simulink model "neuronchainv5"  (Simulink 7.6)
settings: Solver=ode45  StartTime=0.0  StopTime=200  RelTol=1e-3
values from neighbouring files (symbols this model uses):
  alpha = 0.8    [excneuroninit.m]
  beta = 0.05    [excneuroninit.m]
  inittime = 0.1    [excneuroninit.m]
  sensoryamp = 0.5    [excneuroninit.m]
  sigslopef = 1    [excneuroninit.m]
  sigslopei = 3    [excneuroninit.m]
  tau_s = 5    [excneuroninit.m]
libraries: simulink x500, neuronpoolibv3 x3
(part 7 of 18)

== system neuronchainv5/Hebbconp5/44 ==
  ui : Inport
  uj : Inport  Port=2
  Sij : Inport  Port=3
  1_over_taus : Gain  Gain=1/tau_s
  Clock : Clock
      settings: Decimation=10
  Constant : Constant  Value=alpha
  Constant3 : Constant  Value=inittime
  Integrator : Integrator
  Product : Product  Inputs=3  RndMeth=Zero
  Product1 : Product  RndMeth=Zero
  Sum : Sum  Inputs=|+-
  Sum1 : Sum  Inputs=|+-
  Sum2 : Sum  Inputs=+-|
  Switch1 : Switch  Criteria=u2 > Threshold
  beta : Gain  Gain=beta
  f(ui) : Subsystem  TreatAsAtomicUnit=on  mask{slope=sigslopef, offset=0.5}
      mask help: Created by Han, Cheol
      mask Display: plot([10 15 20 25 30 35 40 45 50], [0 0.01 0.1 0.2 0.5 0.8 0.9 0.99 1])
  f(uj) : Subsystem  TreatAsAtomicUnit=on  mask{slope=sigslopef, offset=0.5}
      mask help: Created by Han, Cheol
      mask Display: plot([10 15 20 25 30 35 40 45 50], [0 0.01 0.1 0.2 0.5 0.8 0.9 0.99 1])
  h(ui) : Subsystem  TreatAsAtomicUnit=on  mask{slope=sigslopei, offset=0.5}
      mask help: Created by Han, Cheol
      mask Display: plot([10 15 20 25 30 35 40 45 50], [0 0.01 0.1 0.2 0.5 0.8 0.9 0.99 1])
  Out1 : Outport
  wires:
  ui/1 -> h(ui)/1(x), f(ui)/1(x)
  uj/1 -> f(uj)/1(x)
  f(ui)/1(y) -> Product/1
  f(uj)/1(y) -> Product/2
  Constant/1 -> Product/3
  Product/1 -> Sum/1
  Sum/1 -> Product1/2
  h(ui)/1(y) -> Product1/1
  Product1/1 -> Sum1/1
  beta/1 -> Sum1/2
  Sum1/1 -> 1_over_taus/1
  1_over_taus/1 -> Integrator/1
  Integrator/1 -> Switch1/1, Sum/2
  Sum2/1 -> Switch1/2
  Clock/1 -> Sum2/1
  Constant3/1 -> Sum2/2
  Switch1/1 -> beta/1, Out1/1
  Sij/1 -> Switch1/3

== system neuronchainv5/Hebbconp5/45 ==
  ui : Inport
  uj : Inport  Port=2
  Sij : Inport  Port=3
  1_over_taus : Gain  Gain=1/tau_s
  Clock : Clock
      settings: Decimation=10
  Constant : Constant  Value=alpha
  Constant3 : Constant  Value=inittime
  Integrator : Integrator
  Product : Product  Inputs=3  RndMeth=Zero
  Product1 : Product  RndMeth=Zero
  Sum : Sum  Inputs=|+-
  Sum1 : Sum  Inputs=|+-
  Sum2 : Sum  Inputs=+-|
  Switch1 : Switch  Criteria=u2 > Threshold
  beta : Gain  Gain=beta
  f(ui) : Subsystem  TreatAsAtomicUnit=on  mask{slope=sigslopef, offset=0.5}
      mask help: Created by Han, Cheol
      mask Display: plot([10 15 20 25 30 35 40 45 50], [0 0.01 0.1 0.2 0.5 0.8 0.9 0.99 1])
  f(uj) : Subsystem  TreatAsAtomicUnit=on  mask{slope=sigslopef, offset=0.5}
      mask help: Created by Han, Cheol
      mask Display: plot([10 15 20 25 30 35 40 45 50], [0 0.01 0.1 0.2 0.5 0.8 0.9 0.99 1])
  h(ui) : Subsystem  TreatAsAtomicUnit=on  mask{slope=sigslopei, offset=0.5}
      mask help: Created by Han, Cheol
      mask Display: plot([10 15 20 25 30 35 40 45 50], [0 0.01 0.1 0.2 0.5 0.8 0.9 0.99 1])
  Out1 : Outport
  wires:
  ui/1 -> h(ui)/1(x), f(ui)/1(x)
  uj/1 -> f(uj)/1(x)
  f(ui)/1(y) -> Product/1
  f(uj)/1(y) -> Product/2
  Constant/1 -> Product/3
  Product/1 -> Sum/1
  Sum/1 -> Product1/2
  h(ui)/1(y) -> Product1/1
  Product1/1 -> Sum1/1
  beta/1 -> Sum1/2
  Sum1/1 -> 1_over_taus/1
  1_over_taus/1 -> Integrator/1
  Integrator/1 -> Switch1/1, Sum/2
  Sum2/1 -> Switch1/2
  Clock/1 -> Sum2/1
  Constant3/1 -> Sum2/2
  Switch1/1 -> beta/1, Out1/1
  Sij/1 -> Switch1/3

== system neuronchainv5/Hebbconp5/5 ==
  ui : Inport
  uj : Inport  Port=2
  Sij : Inport  Port=3
  1_over_taus : Gain  Gain=1/tau_s
  Clock : Clock
      settings: Decimation=10
  Constant : Constant  Value=alpha
  Constant3 : Constant  Value=inittime
  Integrator : Integrator
  Product : Product  Inputs=3  RndMeth=Zero
  Product1 : Product  RndMeth=Zero
  Sum : Sum  Inputs=|+-
  Sum1 : Sum  Inputs=|+-
  Sum2 : Sum  Inputs=+-|
  Switch1 : Switch  Criteria=u2 > Threshold
  beta : Gain  Gain=beta
  f(ui) : Subsystem  TreatAsAtomicUnit=on  mask{slope=sigslopef, offset=0.5}
      mask help: Created by Han, Cheol
      mask Display: plot([10 15 20 25 30 35 40 45 50], [0 0.01 0.1 0.2 0.5 0.8 0.9 0.99 1])
  f(uj) : Subsystem  TreatAsAtomicUnit=on  mask{slope=sigslopef, offset=0.5}
      mask help: Created by Han, Cheol
      mask Display: plot([10 15 20 25 30 35 40 45 50], [0 0.01 0.1 0.2 0.5 0.8 0.9 0.99 1])
  h(ui) : Subsystem  TreatAsAtomicUnit=on  mask{slope=sigslopei, offset=0.5}
      mask help: Created by Han, Cheol
      mask Display: plot([10 15 20 25 30 35 40 45 50], [0 0.01 0.1 0.2 0.5 0.8 0.9 0.99 1])
  Out1 : Outport
  wires:
  ui/1 -> h(ui)/1(x), f(ui)/1(x)
  uj/1 -> f(uj)/1(x)
  f(ui)/1(y) -> Product/1
  f(uj)/1(y) -> Product/2
  Constant/1 -> Product/3
  Product/1 -> Sum/1
  Sum/1 -> Product1/2
  h(ui)/1(y) -> Product1/1
  Product1/1 -> Sum1/1
  beta/1 -> Sum1/2
  Sum1/1 -> 1_over_taus/1
  1_over_taus/1 -> Integrator/1
  Integrator/1 -> Switch1/1, Sum/2
  Sum2/1 -> Switch1/2
  Clock/1 -> Sum2/1
  Constant3/1 -> Sum2/2
  Switch1/1 -> beta/1, Out1/1
  Sij/1 -> Switch1/3

== system neuronchainv5/Hebbconp5/f(uj)1 ==
  x : Inport
  Constant : Constant  Value=offset
  Constant1 : Constant  Value=slope
  Constant2 : Constant
  Gain : Gain  Gain=-1  SaturateOnIntegerOverflow=on  OutDataTypeStr=Inherit: Same as input  ParamDataTypeStr=Inherit: Same as input
  Math Function : Math  SaturateOnIntegerOverflow=on
  Math Function1 : Math  Operator=reciprocal  SaturateOnIntegerOverflow=on
  Model Info : simulink/Model-Wide Utilities/Model Info  SystemSampleTime=-1  InitialBlockCM=None  BlockCM=None  Frame=on  DisplayStringWithTags=|  HorizontalTextAlignment=Center  LeftAlignmentValue=0.5  SourceBlockDiagram=neuronchainv5  TagMaxNumber=20
      | Model Info
      | %<Creator> Han, Cheol
  Product : Product  SaturateOnIntegerOverflow=on  OutDataTypeStr=Inherit: Same as first input
  Sum : Sum  Inputs=+-  SaturateOnIntegerOverflow=on
  Sum1 : Sum  SaturateOnIntegerOverflow=on
  y : Outport  InitialOutput=0
  wires:
  x/1 -> Sum/1
  Constant/1 -> Sum/2
  Sum/1 -> Product/1
  Constant1/1 -> Product/2
  Product/1 -> Gain/1
  Gain/1 -> Math Function/1
  Math Function/1 -> Sum1/1
  Constant2/1 -> Sum1/2
  Sum1/1 -> Math Function1/1
  Math Function1/1 -> y/1

== system neuronchainv5/Hebbconp5/f(uj)2 ==
  x : Inport
  Constant : Constant  Value=offset
  Constant1 : Constant  Value=slope
  Constant2 : Constant
  Gain : Gain  Gain=-1  SaturateOnIntegerOverflow=on  OutDataTypeStr=Inherit: Same as input  ParamDataTypeStr=Inherit: Same as input
  Math Function : Math  SaturateOnIntegerOverflow=on
  Math Function1 : Math  Operator=reciprocal  SaturateOnIntegerOverflow=on
  Model Info : simulink/Model-Wide Utilities/Model Info  SystemSampleTime=-1  InitialBlockCM=None  BlockCM=None  Frame=on  DisplayStringWithTags=|  HorizontalTextAlignment=Center  LeftAlignmentValue=0.5  SourceBlockDiagram=neuronchainv5  TagMaxNumber=20
      | Model Info
      | %<Creator> Han, Cheol
  Product : Product  SaturateOnIntegerOverflow=on  OutDataTypeStr=Inherit: Same as first input
  Sum : Sum  Inputs=+-  SaturateOnIntegerOverflow=on
  Sum1 : Sum  SaturateOnIntegerOverflow=on
  y : Outport  InitialOutput=0
  wires:
  x/1 -> Sum/1
  Constant/1 -> Sum/2
  Sum/1 -> Product/1
  Constant1/1 -> Product/2
  Product/1 -> Gain/1
  Gain/1 -> Math Function/1
  Math Function/1 -> Sum1/1
  Constant2/1 -> Sum1/2
  Sum1/1 -> Math Function1/1
  Math Function1/1 -> y/1

== system neuronchainv5/Hebbconp5/f(uj)3 ==
  x : Inport
  Constant : Constant  Value=offset
  Constant1 : Constant  Value=slope
  Constant2 : Constant
  Gain : Gain  Gain=-1  SaturateOnIntegerOverflow=on  OutDataTypeStr=Inherit: Same as input  ParamDataTypeStr=Inherit: Same as input
  Math Function : Math  SaturateOnIntegerOverflow=on
  Math Function1 : Math  Operator=reciprocal  SaturateOnIntegerOverflow=on
  Model Info : simulink/Model-Wide Utilities/Model Info  SystemSampleTime=-1  InitialBlockCM=None  BlockCM=None  Frame=on  DisplayStringWithTags=|  HorizontalTextAlignment=Center  LeftAlignmentValue=0.5  SourceBlockDiagram=neuronchainv5  TagMaxNumber=20
      | Model Info
      | %<Creator> Han, Cheol
  Product : Product  SaturateOnIntegerOverflow=on  OutDataTypeStr=Inherit: Same as first input
  Sum : Sum  Inputs=+-  SaturateOnIntegerOverflow=on
  Sum1 : Sum  SaturateOnIntegerOverflow=on
  y : Outport  InitialOutput=0
  wires:
  x/1 -> Sum/1
  Constant/1 -> Sum/2
  Sum/1 -> Product/1
  Constant1/1 -> Product/2
  Product/1 -> Gain/1
  Gain/1 -> Math Function/1
  Math Function/1 -> Sum1/1
  Constant2/1 -> Sum1/2
  Sum1/1 -> Math Function1/1
  Math Function1/1 -> y/1

== system neuronchainv5/Hebbconp5/f(uj)4 ==
  x : Inport
  Constant : Constant  Value=offset
  Constant1 : Constant  Value=slope
  Constant2 : Constant
  Gain : Gain  Gain=-1  SaturateOnIntegerOverflow=on  OutDataTypeStr=Inherit: Same as input  ParamDataTypeStr=Inherit: Same as input
  Math Function : Math  SaturateOnIntegerOverflow=on
  Math Function1 : Math  Operator=reciprocal  SaturateOnIntegerOverflow=on
  Model Info : simulink/Model-Wide Utilities/Model Info  SystemSampleTime=-1  InitialBlockCM=None  BlockCM=None  Frame=on  DisplayStringWithTags=|  HorizontalTextAlignment=Center  LeftAlignmentValue=0.5  SourceBlockDiagram=neuronchainv5  TagMaxNumber=20
      | Model Info
      | %<Creator> Han, Cheol
  Product : Product  SaturateOnIntegerOverflow=on  OutDataTypeStr=Inherit: Same as first input
  Sum : Sum  Inputs=+-  SaturateOnIntegerOverflow=on
  Sum1 : Sum  SaturateOnIntegerOverflow=on
  y : Outport  InitialOutput=0
  wires:
  x/1 -> Sum/1
  Constant/1 -> Sum/2
  Sum/1 -> Product/1
  Constant1/1 -> Product/2
  Product/1 -> Gain/1
  Gain/1 -> Math Function/1
  Math Function/1 -> Sum1/1
  Constant2/1 -> Sum1/2
  Sum1/1 -> Math Function1/1
  Math Function1/1 -> y/1

== system neuronchainv5/Hebbconp5/f(uj)5 ==
  x : Inport
  Constant : Constant  Value=offset
  Constant1 : Constant  Value=slope
  Constant2 : Constant
  Gain : Gain  Gain=-1  SaturateOnIntegerOverflow=on  OutDataTypeStr=Inherit: Same as input  ParamDataTypeStr=Inherit: Same as input
  Math Function : Math  SaturateOnIntegerOverflow=on
  Math Function1 : Math  Operator=reciprocal  SaturateOnIntegerOverflow=on
  Model Info : simulink/Model-Wide Utilities/Model Info  SystemSampleTime=-1  InitialBlockCM=None  BlockCM=None  Frame=on  DisplayStringWithTags=|  HorizontalTextAlignment=Center  LeftAlignmentValue=0.5  SourceBlockDiagram=neuronchainv5  TagMaxNumber=20
      | Model Info
      | %<Creator> Han, Cheol
  Product : Product  SaturateOnIntegerOverflow=on  OutDataTypeStr=Inherit: Same as first input
  Sum : Sum  Inputs=+-  SaturateOnIntegerOverflow=on
  Sum1 : Sum  SaturateOnIntegerOverflow=on
  y : Outport  InitialOutput=0
  wires:
  x/1 -> Sum/1
  Constant/1 -> Sum/2
  Sum/1 -> Product/1
  Constant1/1 -> Product/2
  Product/1 -> Gain/1
  Gain/1 -> Math Function/1
  Math Function/1 -> Sum1/1
  Constant2/1 -> Sum1/2
  Sum1/1 -> Math Function1/1
  Math Function1/1 -> y/1

== system neuronchainv5/Subsystem/motoract vis inputs ==
  Mux : Mux  Inputs=5
  Mux1 : Mux  Inputs=5
  Subsystem : Subsystem
  Subsystem1 : Subsystem
  Subsystem2 : Subsystem
  Subsystem3 : Subsystem
  Subsystem4 : Subsystem
  Out1 : Outport
  Out2 : Outport  Port=2
  wires:
  Subsystem/1(Out1) -> Mux/1
  Subsystem3/1(Out1) -> Mux/4
  Subsystem/2(Out2) -> Mux1/1
  Subsystem2/2(Out2) -> Mux1/3
  Subsystem3/2(Out2) -> Mux1/4
  Mux/1 -> Out1/1
  Mux1/1 -> Out2/1
  Subsystem1/2(Out2) -> Mux1/2
  Subsystem1/1(Out1) -> Mux/2
  Subsystem2/1(Out1) -> Mux/3
  Subsystem4/2(Out2) -> Mux1/5
  Subsystem4/1(Out1) -> Mux/5

== system neuronchainv5/Hebbconp/ /f(ui) ==
  x : Inport
  Constant : Constant  Value=offset
  Constant1 : Constant  Value=slope
  Constant2 : Constant
  Gain : Gain  Gain=-1  SaturateOnIntegerOverflow=on  OutDataTypeStr=Inherit: Same as input  ParamDataTypeStr=Inherit: Same as input
  Math Function : Math  SaturateOnIntegerOverflow=on
  Math Function1 : Math  Operator=reciprocal  SaturateOnIntegerOverflow=on
  Model Info : simulink/Model-Wide Utilities/Model Info  SystemSampleTime=-1  InitialBlockCM=None  BlockCM=None  Frame=on  DisplayStringWithTags=|  HorizontalTextAlignment=Center  LeftAlignmentValue=0.5  SourceBlockDiagram=neuronchainv5  TagMaxNumber=20
      | Model Info
      | %<Creator> Han, Cheol
  Product : Product  SaturateOnIntegerOverflow=on  OutDataTypeStr=Inherit: Same as first input
  Sum : Sum  Inputs=+-  SaturateOnIntegerOverflow=on
  Sum1 : Sum  SaturateOnIntegerOverflow=on
  y : Outport  InitialOutput=0
  wires:
  x/1 -> Sum/1
  Constant/1 -> Sum/2
  Sum/1 -> Product/1
  Constant1/1 -> Product/2
  Product/1 -> Gain/1
  Gain/1 -> Math Function/1
  Math Function/1 -> Sum1/1
  Constant2/1 -> Sum1/2
  Sum1/1 -> Math Function1/1
  Math Function1/1 -> y/1

== system neuronchainv5/Hebbconp/ /f(uj) ==
  x : Inport
  Constant : Constant  Value=offset
  Constant1 : Constant  Value=slope
  Constant2 : Constant
  Gain : Gain  Gain=-1  SaturateOnIntegerOverflow=on  OutDataTypeStr=Inherit: Same as input  ParamDataTypeStr=Inherit: Same as input
  Math Function : Math  SaturateOnIntegerOverflow=on
  Math Function1 : Math  Operator=reciprocal  SaturateOnIntegerOverflow=on
  Model Info : simulink/Model-Wide Utilities/Model Info  SystemSampleTime=-1  InitialBlockCM=None  BlockCM=None  Frame=on  DisplayStringWithTags=|  HorizontalTextAlignment=Center  LeftAlignmentValue=0.5  SourceBlockDiagram=neuronchainv5  TagMaxNumber=20
      | Model Info
      | %<Creator> Han, Cheol
  Product : Product  SaturateOnIntegerOverflow=on  OutDataTypeStr=Inherit: Same as first input
  Sum : Sum  Inputs=+-  SaturateOnIntegerOverflow=on
  Sum1 : Sum  SaturateOnIntegerOverflow=on
  y : Outport  InitialOutput=0
  wires:
  x/1 -> Sum/1
  Constant/1 -> Sum/2
  Sum/1 -> Product/1
  Constant1/1 -> Product/2
  Product/1 -> Gain/1
  Gain/1 -> Math Function/1
  Math Function/1 -> Sum1/1
  Constant2/1 -> Sum1/2
  Sum1/1 -> Math Function1/1
  Math Function1/1 -> y/1

== system neuronchainv5/Hebbconp/ /h(ui) ==
  x : Inport
  Constant : Constant  Value=offset
  Constant1 : Constant  Value=slope
  Constant2 : Constant
  Gain : Gain  Gain=-1  SaturateOnIntegerOverflow=on  OutDataTypeStr=Inherit: Same as input  ParamDataTypeStr=Inherit: Same as input
  Math Function : Math  SaturateOnIntegerOverflow=on
  Math Function1 : Math  Operator=reciprocal  SaturateOnIntegerOverflow=on
  Model Info : simulink/Model-Wide Utilities/Model Info  SystemSampleTime=-1  InitialBlockCM=None  BlockCM=None  Frame=on  DisplayStringWithTags=|  HorizontalTextAlignment=Center  LeftAlignmentValue=0.5  SourceBlockDiagram=neuronchainv5  TagMaxNumber=20
      | Model Info
      | %<Creator> Han, Cheol
  Product : Product  SaturateOnIntegerOverflow=on  OutDataTypeStr=Inherit: Same as first input
  Sum : Sum  Inputs=+-  SaturateOnIntegerOverflow=on
  Sum1 : Sum  SaturateOnIntegerOverflow=on
  y : Outport  InitialOutput=0
  wires:
  x/1 -> Sum/1
  Constant/1 -> Sum/2
  Sum/1 -> Product/1
  Constant1/1 -> Product/2
  Product/1 -> Gain/1
  Gain/1 -> Math Function/1
  Math Function/1 -> Sum1/1
  Constant2/1 -> Sum1/2
  Sum1/1 -> Math Function1/1
  Math Function1/1 -> y/1

== system neuronchainv5/Hebbconp/ 2/f(ui) ==
  x : Inport
  Constant : Constant  Value=offset
  Constant1 : Constant  Value=slope
  Constant2 : Constant
  Gain : Gain  Gain=-1  SaturateOnIntegerOverflow=on  OutDataTypeStr=Inherit: Same as input  ParamDataTypeStr=Inherit: Same as input
  Math Function : Math  SaturateOnIntegerOverflow=on
  Math Function1 : Math  Operator=reciprocal  SaturateOnIntegerOverflow=on
  Model Info : simulink/Model-Wide Utilities/Model Info  SystemSampleTime=-1  InitialBlockCM=None  BlockCM=None  Frame=on  DisplayStringWithTags=|  HorizontalTextAlignment=Center  LeftAlignmentValue=0.5  SourceBlockDiagram=neuronchainv5  TagMaxNumber=20
      | Model Info
      | %<Creator> Han, Cheol
  Product : Product  SaturateOnIntegerOverflow=on  OutDataTypeStr=Inherit: Same as first input
  Sum : Sum  Inputs=+-  SaturateOnIntegerOverflow=on
  Sum1 : Sum  SaturateOnIntegerOverflow=on
  y : Outport  InitialOutput=0
  wires:
  x/1 -> Sum/1
  Constant/1 -> Sum/2
  Sum/1 -> Product/1
  Constant1/1 -> Product/2
  Product/1 -> Gain/1
  Gain/1 -> Math Function/1
  Math Function/1 -> Sum1/1
  Constant2/1 -> Sum1/2
  Sum1/1 -> Math Function1/1
  Math Function1/1 -> y/1

== system neuronchainv5/Hebbconp/ 2/f(uj) ==
  x : Inport
  Constant : Constant  Value=offset
  Constant1 : Constant  Value=slope
  Constant2 : Constant
  Gain : Gain  Gain=-1  SaturateOnIntegerOverflow=on  OutDataTypeStr=Inherit: Same as input  ParamDataTypeStr=Inherit: Same as input
  Math Function : Math  SaturateOnIntegerOverflow=on
  Math Function1 : Math  Operator=reciprocal  SaturateOnIntegerOverflow=on
  Model Info : simulink/Model-Wide Utilities/Model Info  SystemSampleTime=-1  InitialBlockCM=None  BlockCM=None  Frame=on  DisplayStringWithTags=|  HorizontalTextAlignment=Center  LeftAlignmentValue=0.5  SourceBlockDiagram=neuronchainv5  TagMaxNumber=20
      | Model Info
      | %<Creator> Han, Cheol
  Product : Product  SaturateOnIntegerOverflow=on  OutDataTypeStr=Inherit: Same as first input
  Sum : Sum  Inputs=+-  SaturateOnIntegerOverflow=on
  Sum1 : Sum  SaturateOnIntegerOverflow=on
  y : Outport  InitialOutput=0
  wires:
  x/1 -> Sum/1
  Constant/1 -> Sum/2
  Sum/1 -> Product/1
  Constant1/1 -> Product/2
  Product/1 -> Gain/1
  Gain/1 -> Math Function/1
  Math Function/1 -> Sum1/1
  Constant2/1 -> Sum1/2
  Sum1/1 -> Math Function1/1
  Math Function1/1 -> y/1

== system neuronchainv5/Hebbconp/ 2/h(ui) ==
  x : Inport
  Constant : Constant  Value=offset
  Constant1 : Constant  Value=slope
  Constant2 : Constant
  Gain : Gain  Gain=-1  SaturateOnIntegerOverflow=on  OutDataTypeStr=Inherit: Same as input  ParamDataTypeStr=Inherit: Same as input
  Math Function : Math  SaturateOnIntegerOverflow=on
  Math Function1 : Math  Operator=reciprocal  SaturateOnIntegerOverflow=on
  Model Info : simulink/Model-Wide Utilities/Model Info  SystemSampleTime=-1  InitialBlockCM=None  BlockCM=None  Frame=on  DisplayStringWithTags=|  HorizontalTextAlignment=Center  LeftAlignmentValue=0.5  SourceBlockDiagram=neuronchainv5  TagMaxNumber=20
      | Model Info
      | %<Creator> Han, Cheol
  Product : Product  SaturateOnIntegerOverflow=on  OutDataTypeStr=Inherit: Same as first input
  Sum : Sum  Inputs=+-  SaturateOnIntegerOverflow=on
  Sum1 : Sum  SaturateOnIntegerOverflow=on
  y : Outport  InitialOutput=0
  wires:
  x/1 -> Sum/1
  Constant/1 -> Sum/2
  Sum/1 -> Product/1
  Constant1/1 -> Product/2
  Product/1 -> Gain/1
  Gain/1 -> Math Function/1
  Math Function/1 -> Sum1/1
  Constant2/1 -> Sum1/2
  Sum1/1 -> Math Function1/1
  Math Function1/1 -> y/1

== system neuronchainv5/Hebbconp/11/f(ui) ==
  x : Inport
  Constant : Constant  Value=offset
  Constant1 : Constant  Value=slope
  Constant2 : Constant
  Gain : Gain  Gain=-1  SaturateOnIntegerOverflow=on  OutDataTypeStr=Inherit: Same as input  ParamDataTypeStr=Inherit: Same as input
  Math Function : Math  SaturateOnIntegerOverflow=on
  Math Function1 : Math  Operator=reciprocal  SaturateOnIntegerOverflow=on
  Model Info : simulink/Model-Wide Utilities/Model Info  SystemSampleTime=-1  InitialBlockCM=None  BlockCM=None  Frame=on  DisplayStringWithTags=|  HorizontalTextAlignment=Center  LeftAlignmentValue=0.5  SourceBlockDiagram=neuronchainv5  TagMaxNumber=20
      | Model Info
      | %<Creator> Han, Cheol
  Product : Product  SaturateOnIntegerOverflow=on  OutDataTypeStr=Inherit: Same as first input
  Sum : Sum  Inputs=+-  SaturateOnIntegerOverflow=on
  Sum1 : Sum  SaturateOnIntegerOverflow=on
  y : Outport  InitialOutput=0
  wires:
  x/1 -> Sum/1
  Constant/1 -> Sum/2
  Sum/1 -> Product/1
  Constant1/1 -> Product/2
  Product/1 -> Gain/1
  Gain/1 -> Math Function/1
  Math Function/1 -> Sum1/1
  Constant2/1 -> Sum1/2
  Sum1/1 -> Math Function1/1
  Math Function1/1 -> y/1

== system neuronchainv5/Hebbconp/11/f(uj) ==
  x : Inport
  Constant : Constant  Value=offset
  Constant1 : Constant  Value=slope
  Constant2 : Constant
  Gain : Gain  Gain=-1  SaturateOnIntegerOverflow=on  OutDataTypeStr=Inherit: Same as input  ParamDataTypeStr=Inherit: Same as input
  Math Function : Math  SaturateOnIntegerOverflow=on
  Math Function1 : Math  Operator=reciprocal  SaturateOnIntegerOverflow=on
  Model Info : simulink/Model-Wide Utilities/Model Info  SystemSampleTime=-1  InitialBlockCM=None  BlockCM=None  Frame=on  DisplayStringWithTags=|  HorizontalTextAlignment=Center  LeftAlignmentValue=0.5  SourceBlockDiagram=neuronchainv5  TagMaxNumber=20
      | Model Info
      | %<Creator> Han, Cheol
  Product : Product  SaturateOnIntegerOverflow=on  OutDataTypeStr=Inherit: Same as first input
  Sum : Sum  Inputs=+-  SaturateOnIntegerOverflow=on
  Sum1 : Sum  SaturateOnIntegerOverflow=on
  y : Outport  InitialOutput=0
  wires:
  x/1 -> Sum/1
  Constant/1 -> Sum/2
  Sum/1 -> Product/1
  Constant1/1 -> Product/2
  Product/1 -> Gain/1
  Gain/1 -> Math Function/1
  Math Function/1 -> Sum1/1
  Constant2/1 -> Sum1/2
  Sum1/1 -> Math Function1/1
  Math Function1/1 -> y/1

== system neuronchainv5/Hebbconp/11/h(ui) ==
  x : Inport
  Constant : Constant  Value=offset
  Constant1 : Constant  Value=slope
  Constant2 : Constant
  Gain : Gain  Gain=-1  SaturateOnIntegerOverflow=on  OutDataTypeStr=Inherit: Same as input  ParamDataTypeStr=Inherit: Same as input
  Math Function : Math  SaturateOnIntegerOverflow=on
  Math Function1 : Math  Operator=reciprocal  SaturateOnIntegerOverflow=on
  Model Info : simulink/Model-Wide Utilities/Model Info  SystemSampleTime=-1  InitialBlockCM=None  BlockCM=None  Frame=on  DisplayStringWithTags=|  HorizontalTextAlignment=Center  LeftAlignmentValue=0.5  SourceBlockDiagram=neuronchainv5  TagMaxNumber=20
      | Model Info
      | %<Creator> Han, Cheol
  Product : Product  SaturateOnIntegerOverflow=on  OutDataTypeStr=Inherit: Same as first input
  Sum : Sum  Inputs=+-  SaturateOnIntegerOverflow=on
  Sum1 : Sum  SaturateOnIntegerOverflow=on
  y : Outport  InitialOutput=0
  wires:
  x/1 -> Sum/1
  Constant/1 -> Sum/2
  Sum/1 -> Product/1
  Constant1/1 -> Product/2
  Product/1 -> Gain/1
  Gain/1 -> Math Function/1
  Math Function/1 -> Sum1/1
  Constant2/1 -> Sum1/2
  Sum1/1 -> Math Function1/1
  Math Function1/1 -> y/1

== system neuronchainv5/Hebbconp/12/f(ui) ==
  x : Inport
  Constant : Constant  Value=offset
  Constant1 : Constant  Value=slope
  Constant2 : Constant
  Gain : Gain  Gain=-1  SaturateOnIntegerOverflow=on  OutDataTypeStr=Inherit: Same as input  ParamDataTypeStr=Inherit: Same as input
  Math Function : Math  SaturateOnIntegerOverflow=on
  Math Function1 : Math  Operator=reciprocal  SaturateOnIntegerOverflow=on
  Model Info : simulink/Model-Wide Utilities/Model Info  SystemSampleTime=-1  InitialBlockCM=None  BlockCM=None  Frame=on  DisplayStringWithTags=|  HorizontalTextAlignment=Center  LeftAlignmentValue=0.5  SourceBlockDiagram=neuronchainv5  TagMaxNumber=20
      | Model Info
      | %<Creator> Han, Cheol
  Product : Product  SaturateOnIntegerOverflow=on  OutDataTypeStr=Inherit: Same as first input
  Sum : Sum  Inputs=+-  SaturateOnIntegerOverflow=on
  Sum1 : Sum  SaturateOnIntegerOverflow=on
  y : Outport  InitialOutput=0
  wires:
  x/1 -> Sum/1
  Constant/1 -> Sum/2
  Sum/1 -> Product/1
  Constant1/1 -> Product/2
  Product/1 -> Gain/1
  Gain/1 -> Math Function/1
  Math Function/1 -> Sum1/1
  Constant2/1 -> Sum1/2
  Sum1/1 -> Math Function1/1
  Math Function1/1 -> y/1

== system neuronchainv5/Hebbconp/12/f(uj) ==
  x : Inport
  Constant : Constant  Value=offset
  Constant1 : Constant  Value=slope
  Constant2 : Constant
  Gain : Gain  Gain=-1  SaturateOnIntegerOverflow=on  OutDataTypeStr=Inherit: Same as input  ParamDataTypeStr=Inherit: Same as input
  Math Function : Math  SaturateOnIntegerOverflow=on
  Math Function1 : Math  Operator=reciprocal  SaturateOnIntegerOverflow=on
  Model Info : simulink/Model-Wide Utilities/Model Info  SystemSampleTime=-1  InitialBlockCM=None  BlockCM=None  Frame=on  DisplayStringWithTags=|  HorizontalTextAlignment=Center  LeftAlignmentValue=0.5  SourceBlockDiagram=neuronchainv5  TagMaxNumber=20
      | Model Info
      | %<Creator> Han, Cheol
  Product : Product  SaturateOnIntegerOverflow=on  OutDataTypeStr=Inherit: Same as first input
  Sum : Sum  Inputs=+-  SaturateOnIntegerOverflow=on
  Sum1 : Sum  SaturateOnIntegerOverflow=on
  y : Outport  InitialOutput=0
  wires:
  x/1 -> Sum/1
  Constant/1 -> Sum/2
  Sum/1 -> Product/1
  Constant1/1 -> Product/2
  Product/1 -> Gain/1
  Gain/1 -> Math Function/1
  Math Function/1 -> Sum1/1
  Constant2/1 -> Sum1/2
  Sum1/1 -> Math Function1/1
  Math Function1/1 -> y/1

== system neuronchainv5/Hebbconp/12/h(ui) ==
  x : Inport
  Constant : Constant  Value=offset
  Constant1 : Constant  Value=slope
  Constant2 : Constant
  Gain : Gain  Gain=-1  SaturateOnIntegerOverflow=on  OutDataTypeStr=Inherit: Same as input  ParamDataTypeStr=Inherit: Same as input
  Math Function : Math  SaturateOnIntegerOverflow=on
  Math Function1 : Math  Operator=reciprocal  SaturateOnIntegerOverflow=on
  Model Info : simulink/Model-Wide Utilities/Model Info  SystemSampleTime=-1  InitialBlockCM=None  BlockCM=None  Frame=on  DisplayStringWithTags=|  HorizontalTextAlignment=Center  LeftAlignmentValue=0.5  SourceBlockDiagram=neuronchainv5  TagMaxNumber=20
      | Model Info
      | %<Creator> Han, Cheol
  Product : Product  SaturateOnIntegerOverflow=on  OutDataTypeStr=Inherit: Same as first input
  Sum : Sum  Inputs=+-  SaturateOnIntegerOverflow=on
  Sum1 : Sum  SaturateOnIntegerOverflow=on
  y : Outport  InitialOutput=0
  wires:
  x/1 -> Sum/1
  Constant/1 -> Sum/2
  Sum/1 -> Product/1
  Constant1/1 -> Product/2
  Product/1 -> Gain/1
  Gain/1 -> Math Function/1
  Math Function/1 -> Sum1/1
  Constant2/1 -> Sum1/2
  Sum1/1 -> Math Function1/1
  Math Function1/1 -> y/1

== system neuronchainv5/Hebbconp/13/f(ui) ==
  x : Inport
  Constant : Constant  Value=offset
  Constant1 : Constant  Value=slope
  Constant2 : Constant
  Gain : Gain  Gain=-1  SaturateOnIntegerOverflow=on  OutDataTypeStr=Inherit: Same as input  ParamDataTypeStr=Inherit: Same as input
  Math Function : Math  SaturateOnIntegerOverflow=on
  Math Function1 : Math  Operator=reciprocal  SaturateOnIntegerOverflow=on
  Model Info : simulink/Model-Wide Utilities/Model Info  SystemSampleTime=-1  InitialBlockCM=None  BlockCM=None  Frame=on  DisplayStringWithTags=|  HorizontalTextAlignment=Center  LeftAlignmentValue=0.5  SourceBlockDiagram=neuronchainv5  TagMaxNumber=20
      | Model Info
      | %<Creator> Han, Cheol
  Product : Product  SaturateOnIntegerOverflow=on  OutDataTypeStr=Inherit: Same as first input
  Sum : Sum  Inputs=+-  SaturateOnIntegerOverflow=on
  Sum1 : Sum  SaturateOnIntegerOverflow=on
  y : Outport  InitialOutput=0
  wires:
  x/1 -> Sum/1
  Constant/1 -> Sum/2
  Sum/1 -> Product/1
  Constant1/1 -> Product/2
  Product/1 -> Gain/1
  Gain/1 -> Math Function/1
  Math Function/1 -> Sum1/1
  Constant2/1 -> Sum1/2
  Sum1/1 -> Math Function1/1
  Math Function1/1 -> y/1

== system neuronchainv5/Hebbconp/13/f(uj) ==
  x : Inport
  Constant : Constant  Value=offset
  Constant1 : Constant  Value=slope
  Constant2 : Constant
  Gain : Gain  Gain=-1  SaturateOnIntegerOverflow=on  OutDataTypeStr=Inherit: Same as input  ParamDataTypeStr=Inherit: Same as input
  Math Function : Math  SaturateOnIntegerOverflow=on
  Math Function1 : Math  Operator=reciprocal  SaturateOnIntegerOverflow=on
  Model Info : simulink/Model-Wide Utilities/Model Info  SystemSampleTime=-1  InitialBlockCM=None  BlockCM=None  Frame=on  DisplayStringWithTags=|  HorizontalTextAlignment=Center  LeftAlignmentValue=0.5  SourceBlockDiagram=neuronchainv5  TagMaxNumber=20
      | Model Info
      | %<Creator> Han, Cheol
  Product : Product  SaturateOnIntegerOverflow=on  OutDataTypeStr=Inherit: Same as first input
  Sum : Sum  Inputs=+-  SaturateOnIntegerOverflow=on
  Sum1 : Sum  SaturateOnIntegerOverflow=on
  y : Outport  InitialOutput=0
  wires:
  x/1 -> Sum/1
  Constant/1 -> Sum/2
  Sum/1 -> Product/1
  Constant1/1 -> Product/2
  Product/1 -> Gain/1
  Gain/1 -> Math Function/1
  Math Function/1 -> Sum1/1
  Constant2/1 -> Sum1/2
  Sum1/1 -> Math Function1/1
  Math Function1/1 -> y/1

== system neuronchainv5/Hebbconp/13/h(ui) ==
  x : Inport
  Constant : Constant  Value=offset
  Constant1 : Constant  Value=slope
  Constant2 : Constant
  Gain : Gain  Gain=-1  SaturateOnIntegerOverflow=on  OutDataTypeStr=Inherit: Same as input  ParamDataTypeStr=Inherit: Same as input
  Math Function : Math  SaturateOnIntegerOverflow=on
  Math Function1 : Math  Operator=reciprocal  SaturateOnIntegerOverflow=on
  Model Info : simulink/Model-Wide Utilities/Model Info  SystemSampleTime=-1  InitialBlockCM=None  BlockCM=None  Frame=on  DisplayStringWithTags=|  HorizontalTextAlignment=Center  LeftAlignmentValue=0.5  SourceBlockDiagram=neuronchainv5  TagMaxNumber=20
      | Model Info
      | %<Creator> Han, Cheol
  Product : Product  SaturateOnIntegerOverflow=on  OutDataTypeStr=Inherit: Same as first input
  Sum : Sum  Inputs=+-  SaturateOnIntegerOverflow=on
  Sum1 : Sum  SaturateOnIntegerOverflow=on
  y : Outport  InitialOutput=0
  wires:
  x/1 -> Sum/1
  Constant/1 -> Sum/2
  Sum/1 -> Product/1
  Constant1/1 -> Product/2
  Product/1 -> Gain/1
  Gain/1 -> Math Function/1
  Math Function/1 -> Sum1/1
  Constant2/1 -> Sum1/2
  Sum1/1 -> Math Function1/1
  Math Function1/1 -> y/1

== system neuronchainv5/Hebbconp/14/f(ui) ==
  x : Inport
  Constant : Constant  Value=offset
  Constant1 : Constant  Value=slope
  Constant2 : Constant
  Gain : Gain  Gain=-1  SaturateOnIntegerOverflow=on  OutDataTypeStr=Inherit: Same as input  ParamDataTypeStr=Inherit: Same as input
  Math Function : Math  SaturateOnIntegerOverflow=on
  Math Function1 : Math  Operator=reciprocal  SaturateOnIntegerOverflow=on
  Model Info : simulink/Model-Wide Utilities/Model Info  SystemSampleTime=-1  InitialBlockCM=None  BlockCM=None  Frame=on  DisplayStringWithTags=|  HorizontalTextAlignment=Center  LeftAlignmentValue=0.5  SourceBlockDiagram=neuronchainv5  TagMaxNumber=20
      | Model Info
      | %<Creator> Han, Cheol
  Product : Product  SaturateOnIntegerOverflow=on  OutDataTypeStr=Inherit: Same as first input
  Sum : Sum  Inputs=+-  SaturateOnIntegerOverflow=on
  Sum1 : Sum  SaturateOnIntegerOverflow=on
  y : Outport  InitialOutput=0
  wires:
  x/1 -> Sum/1
  Constant/1 -> Sum/2
  Sum/1 -> Product/1
  Constant1/1 -> Product/2
  Product/1 -> Gain/1
  Gain/1 -> Math Function/1
  Math Function/1 -> Sum1/1
  Constant2/1 -> Sum1/2
  Sum1/1 -> Math Function1/1
  Math Function1/1 -> y/1

== system neuronchainv5/Hebbconp/14/f(uj) ==
  x : Inport
  Constant : Constant  Value=offset
  Constant1 : Constant  Value=slope
  Constant2 : Constant
  Gain : Gain  Gain=-1  SaturateOnIntegerOverflow=on  OutDataTypeStr=Inherit: Same as input  ParamDataTypeStr=Inherit: Same as input
  Math Function : Math  SaturateOnIntegerOverflow=on
  Math Function1 : Math  Operator=reciprocal  SaturateOnIntegerOverflow=on
  Model Info : simulink/Model-Wide Utilities/Model Info  SystemSampleTime=-1  InitialBlockCM=None  BlockCM=None  Frame=on  DisplayStringWithTags=|  HorizontalTextAlignment=Center  LeftAlignmentValue=0.5  SourceBlockDiagram=neuronchainv5  TagMaxNumber=20
      | Model Info
      | %<Creator> Han, Cheol
  Product : Product  SaturateOnIntegerOverflow=on  OutDataTypeStr=Inherit: Same as first input
  Sum : Sum  Inputs=+-  SaturateOnIntegerOverflow=on
  Sum1 : Sum  SaturateOnIntegerOverflow=on
  y : Outport  InitialOutput=0
  wires:
  x/1 -> Sum/1
  Constant/1 -> Sum/2
  Sum/1 -> Product/1
  Constant1/1 -> Product/2
  Product/1 -> Gain/1
  Gain/1 -> Math Function/1
  Math Function/1 -> Sum1/1
  Constant2/1 -> Sum1/2
  Sum1/1 -> Math Function1/1
  Math Function1/1 -> y/1

== system neuronchainv5/Hebbconp/14/h(ui) ==
  x : Inport
  Constant : Constant  Value=offset
  Constant1 : Constant  Value=slope
  Constant2 : Constant
  Gain : Gain  Gain=-1  SaturateOnIntegerOverflow=on  OutDataTypeStr=Inherit: Same as input  ParamDataTypeStr=Inherit: Same as input
  Math Function : Math  SaturateOnIntegerOverflow=on
  Math Function1 : Math  Operator=reciprocal  SaturateOnIntegerOverflow=on
  Model Info : simulink/Model-Wide Utilities/Model Info  SystemSampleTime=-1  InitialBlockCM=None  BlockCM=None  Frame=on  DisplayStringWithTags=|  HorizontalTextAlignment=Center  LeftAlignmentValue=0.5  SourceBlockDiagram=neuronchainv5  TagMaxNumber=20
      | Model Info
      | %<Creator> Han, Cheol
  Product : Product  SaturateOnIntegerOverflow=on  OutDataTypeStr=Inherit: Same as first input
  Sum : Sum  Inputs=+-  SaturateOnIntegerOverflow=on
  Sum1 : Sum  SaturateOnIntegerOverflow=on
  y : Outport  InitialOutput=0
  wires:
  x/1 -> Sum/1
  Constant/1 -> Sum/2
  Sum/1 -> Product/1
  Constant1/1 -> Product/2
  Product/1 -> Gain/1
  Gain/1 -> Math Function/1
  Math Function/1 -> Sum1/1
  Constant2/1 -> Sum1/2
  Sum1/1 -> Math Function1/1
  Math Function1/1 -> y/1

== system neuronchainv5/Hebbconp/15/f(ui) ==
  x : Inport
  Constant : Constant  Value=offset
  Constant1 : Constant  Value=slope
  Constant2 : Constant
  Gain : Gain  Gain=-1  SaturateOnIntegerOverflow=on  OutDataTypeStr=Inherit: Same as input  ParamDataTypeStr=Inherit: Same as input
  Math Function : Math  SaturateOnIntegerOverflow=on
  Math Function1 : Math  Operator=reciprocal  SaturateOnIntegerOverflow=on
  Model Info : simulink/Model-Wide Utilities/Model Info  SystemSampleTime=-1  InitialBlockCM=None  BlockCM=None  Frame=on  DisplayStringWithTags=|  HorizontalTextAlignment=Center  LeftAlignmentValue=0.5  SourceBlockDiagram=neuronchainv5  TagMaxNumber=20
      | Model Info
      | %<Creator> Han, Cheol
  Product : Product  SaturateOnIntegerOverflow=on  OutDataTypeStr=Inherit: Same as first input
  Sum : Sum  Inputs=+-  SaturateOnIntegerOverflow=on
  Sum1 : Sum  SaturateOnIntegerOverflow=on
  y : Outport  InitialOutput=0
  wires:
  x/1 -> Sum/1
  Constant/1 -> Sum/2
  Sum/1 -> Product/1
  Constant1/1 -> Product/2
  Product/1 -> Gain/1
  Gain/1 -> Math Function/1
  Math Function/1 -> Sum1/1
  Constant2/1 -> Sum1/2
  Sum1/1 -> Math Function1/1
  Math Function1/1 -> y/1

== system neuronchainv5/Hebbconp/15/f(uj) ==
  x : Inport
  Constant : Constant  Value=offset
  Constant1 : Constant  Value=slope
  Constant2 : Constant
  Gain : Gain  Gain=-1  SaturateOnIntegerOverflow=on  OutDataTypeStr=Inherit: Same as input  ParamDataTypeStr=Inherit: Same as input
  Math Function : Math  SaturateOnIntegerOverflow=on
  Math Function1 : Math  Operator=reciprocal  SaturateOnIntegerOverflow=on
  Model Info : simulink/Model-Wide Utilities/Model Info  SystemSampleTime=-1  InitialBlockCM=None  BlockCM=None  Frame=on  DisplayStringWithTags=|  HorizontalTextAlignment=Center  LeftAlignmentValue=0.5  SourceBlockDiagram=neuronchainv5  TagMaxNumber=20
      | Model Info
      | %<Creator> Han, Cheol
  Product : Product  SaturateOnIntegerOverflow=on  OutDataTypeStr=Inherit: Same as first input
  Sum : Sum  Inputs=+-  SaturateOnIntegerOverflow=on
  Sum1 : Sum  SaturateOnIntegerOverflow=on
  y : Outport  InitialOutput=0
  wires:
  x/1 -> Sum/1
  Constant/1 -> Sum/2
  Sum/1 -> Product/1
  Constant1/1 -> Product/2
  Product/1 -> Gain/1
  Gain/1 -> Math Function/1
  Math Function/1 -> Sum1/1
  Constant2/1 -> Sum1/2
  Sum1/1 -> Math Function1/1
  Math Function1/1 -> y/1

== system neuronchainv5/Hebbconp/15/h(ui) ==
  x : Inport
  Constant : Constant  Value=offset
  Constant1 : Constant  Value=slope
  Constant2 : Constant
  Gain : Gain  Gain=-1  SaturateOnIntegerOverflow=on  OutDataTypeStr=Inherit: Same as input  ParamDataTypeStr=Inherit: Same as input
  Math Function : Math  SaturateOnIntegerOverflow=on
  Math Function1 : Math  Operator=reciprocal  SaturateOnIntegerOverflow=on
  Model Info : simulink/Model-Wide Utilities/Model Info  SystemSampleTime=-1  InitialBlockCM=None  BlockCM=None  Frame=on  DisplayStringWithTags=|  HorizontalTextAlignment=Center  LeftAlignmentValue=0.5  SourceBlockDiagram=neuronchainv5  TagMaxNumber=20
      | Model Info
      | %<Creator> Han, Cheol
  Product : Product  SaturateOnIntegerOverflow=on  OutDataTypeStr=Inherit: Same as first input
  Sum : Sum  Inputs=+-  SaturateOnIntegerOverflow=on
  Sum1 : Sum  SaturateOnIntegerOverflow=on
  y : Outport  InitialOutput=0
  wires:
  x/1 -> Sum/1
  Constant/1 -> Sum/2
  Sum/1 -> Product/1
  Constant1/1 -> Product/2
  Product/1 -> Gain/1
  Gain/1 -> Math Function/1
  Math Function/1 -> Sum1/1
  Constant2/1 -> Sum1/2
  Sum1/1 -> Math Function1/1
  Math Function1/1 -> y/1

== system neuronchainv5/Hebbconp/21/f(ui) ==
  x : Inport
  Constant : Constant  Value=offset
  Constant1 : Constant  Value=slope
  Constant2 : Constant
  Gain : Gain  Gain=-1  SaturateOnIntegerOverflow=on  OutDataTypeStr=Inherit: Same as input  ParamDataTypeStr=Inherit: Same as input
  Math Function : Math  SaturateOnIntegerOverflow=on
  Math Function1 : Math  Operator=reciprocal  SaturateOnIntegerOverflow=on
  Model Info : simulink/Model-Wide Utilities/Model Info  SystemSampleTime=-1  InitialBlockCM=None  BlockCM=None  Frame=on  DisplayStringWithTags=|  HorizontalTextAlignment=Center  LeftAlignmentValue=0.5  SourceBlockDiagram=neuronchainv5  TagMaxNumber=20
      | Model Info
      | %<Creator> Han, Cheol
  Product : Product  SaturateOnIntegerOverflow=on  OutDataTypeStr=Inherit: Same as first input
  Sum : Sum  Inputs=+-  SaturateOnIntegerOverflow=on
  Sum1 : Sum  SaturateOnIntegerOverflow=on
  y : Outport  InitialOutput=0
  wires:
  x/1 -> Sum/1
  Constant/1 -> Sum/2
  Sum/1 -> Product/1
  Constant1/1 -> Product/2
  Product/1 -> Gain/1
  Gain/1 -> Math Function/1
  Math Function/1 -> Sum1/1
  Constant2/1 -> Sum1/2
  Sum1/1 -> Math Function1/1
  Math Function1/1 -> y/1

== system neuronchainv5/Hebbconp/21/f(uj) ==
  x : Inport
  Constant : Constant  Value=offset
  Constant1 : Constant  Value=slope
  Constant2 : Constant
  Gain : Gain  Gain=-1  SaturateOnIntegerOverflow=on  OutDataTypeStr=Inherit: Same as input  ParamDataTypeStr=Inherit: Same as input
  Math Function : Math  SaturateOnIntegerOverflow=on
  Math Function1 : Math  Operator=reciprocal  SaturateOnIntegerOverflow=on
  Model Info : simulink/Model-Wide Utilities/Model Info  SystemSampleTime=-1  InitialBlockCM=None  BlockCM=None  Frame=on  DisplayStringWithTags=|  HorizontalTextAlignment=Center  LeftAlignmentValue=0.5  SourceBlockDiagram=neuronchainv5  TagMaxNumber=20
      | Model Info
      | %<Creator> Han, Cheol
  Product : Product  SaturateOnIntegerOverflow=on  OutDataTypeStr=Inherit: Same as first input
  Sum : Sum  Inputs=+-  SaturateOnIntegerOverflow=on
  Sum1 : Sum  SaturateOnIntegerOverflow=on
  y : Outport  InitialOutput=0
  wires:
  x/1 -> Sum/1
  Constant/1 -> Sum/2
  Sum/1 -> Product/1
  Constant1/1 -> Product/2
  Product/1 -> Gain/1
  Gain/1 -> Math Function/1
  Math Function/1 -> Sum1/1
  Constant2/1 -> Sum1/2
  Sum1/1 -> Math Function1/1
  Math Function1/1 -> y/1

== system neuronchainv5/Hebbconp/21/h(ui) ==
  x : Inport
  Constant : Constant  Value=offset
  Constant1 : Constant  Value=slope
  Constant2 : Constant
  Gain : Gain  Gain=-1  SaturateOnIntegerOverflow=on  OutDataTypeStr=Inherit: Same as input  ParamDataTypeStr=Inherit: Same as input
  Math Function : Math  SaturateOnIntegerOverflow=on
  Math Function1 : Math  Operator=reciprocal  SaturateOnIntegerOverflow=on
  Model Info : simulink/Model-Wide Utilities/Model Info  SystemSampleTime=-1  InitialBlockCM=None  BlockCM=None  Frame=on  DisplayStringWithTags=|  HorizontalTextAlignment=Center  LeftAlignmentValue=0.5  SourceBlockDiagram=neuronchainv5  TagMaxNumber=20
      | Model Info
      | %<Creator> Han, Cheol
  Product : Product  SaturateOnIntegerOverflow=on  OutDataTypeStr=Inherit: Same as first input
  Sum : Sum  Inputs=+-  SaturateOnIntegerOverflow=on
  Sum1 : Sum  SaturateOnIntegerOverflow=on
  y : Outport  InitialOutput=0
  wires:
  x/1 -> Sum/1
  Constant/1 -> Sum/2
  Sum/1 -> Product/1
  Constant1/1 -> Product/2
  Product/1 -> Gain/1
  Gain/1 -> Math Function/1
  Math Function/1 -> Sum1/1
  Constant2/1 -> Sum1/2
  Sum1/1 -> Math Function1/1
  Math Function1/1 -> y/1

== system neuronchainv5/Hebbconp/22/f(ui) ==
  x : Inport
  Constant : Constant  Value=offset
  Constant1 : Constant  Value=slope
  Constant2 : Constant
  Gain : Gain  Gain=-1  SaturateOnIntegerOverflow=on  OutDataTypeStr=Inherit: Same as input  ParamDataTypeStr=Inherit: Same as input
  Math Function : Math  SaturateOnIntegerOverflow=on
  Math Function1 : Math  Operator=reciprocal  SaturateOnIntegerOverflow=on
  Model Info : simulink/Model-Wide Utilities/Model Info  SystemSampleTime=-1  InitialBlockCM=None  BlockCM=None  Frame=on  DisplayStringWithTags=|  HorizontalTextAlignment=Center  LeftAlignmentValue=0.5  SourceBlockDiagram=neuronchainv5  TagMaxNumber=20
      | Model Info
      | %<Creator> Han, Cheol
  Product : Product  SaturateOnIntegerOverflow=on  OutDataTypeStr=Inherit: Same as first input
  Sum : Sum  Inputs=+-  SaturateOnIntegerOverflow=on
  Sum1 : Sum  SaturateOnIntegerOverflow=on
  y : Outport  InitialOutput=0
  wires:
  x/1 -> Sum/1
  Constant/1 -> Sum/2
  Sum/1 -> Product/1
  Constant1/1 -> Product/2
  Product/1 -> Gain/1
  Gain/1 -> Math Function/1
  Math Function/1 -> Sum1/1
  Constant2/1 -> Sum1/2
  Sum1/1 -> Math Function1/1
  Math Function1/1 -> y/1

== system neuronchainv5/Hebbconp/22/f(uj) ==
  x : Inport
  Constant : Constant  Value=offset
  Constant1 : Constant  Value=slope
  Constant2 : Constant
  Gain : Gain  Gain=-1  SaturateOnIntegerOverflow=on  OutDataTypeStr=Inherit: Same as input  ParamDataTypeStr=Inherit: Same as input
  Math Function : Math  SaturateOnIntegerOverflow=on
  Math Function1 : Math  Operator=reciprocal  SaturateOnIntegerOverflow=on
  Model Info : simulink/Model-Wide Utilities/Model Info  SystemSampleTime=-1  InitialBlockCM=None  BlockCM=None  Frame=on  DisplayStringWithTags=|  HorizontalTextAlignment=Center  LeftAlignmentValue=0.5  SourceBlockDiagram=neuronchainv5  TagMaxNumber=20
      | Model Info
      | %<Creator> Han, Cheol
  Product : Product  SaturateOnIntegerOverflow=on  OutDataTypeStr=Inherit: Same as first input
  Sum : Sum  Inputs=+-  SaturateOnIntegerOverflow=on
  Sum1 : Sum  SaturateOnIntegerOverflow=on
  y : Outport  InitialOutput=0
  wires:
  x/1 -> Sum/1
  Constant/1 -> Sum/2
  Sum/1 -> Product/1
  Constant1/1 -> Product/2
  Product/1 -> Gain/1
  Gain/1 -> Math Function/1
  Math Function/1 -> Sum1/1
  Constant2/1 -> Sum1/2
  Sum1/1 -> Math Function1/1
  Math Function1/1 -> y/1

== system neuronchainv5/Hebbconp/22/h(ui) ==
  x : Inport
  Constant : Constant  Value=offset
  Constant1 : Constant  Value=slope
  Constant2 : Constant
  Gain : Gain  Gain=-1  SaturateOnIntegerOverflow=on  OutDataTypeStr=Inherit: Same as input  ParamDataTypeStr=Inherit: Same as input
  Math Function : Math  SaturateOnIntegerOverflow=on
  Math Function1 : Math  Operator=reciprocal  SaturateOnIntegerOverflow=on
  Model Info : simulink/Model-Wide Utilities/Model Info  SystemSampleTime=-1  InitialBlockCM=None  BlockCM=None  Frame=on  DisplayStringWithTags=|  HorizontalTextAlignment=Center  LeftAlignmentValue=0.5  SourceBlockDiagram=neuronchainv5  TagMaxNumber=20
      | Model Info
      | %<Creator> Han, Cheol
  Product : Product  SaturateOnIntegerOverflow=on  OutDataTypeStr=Inherit: Same as first input
  Sum : Sum  Inputs=+-  SaturateOnIntegerOverflow=on
  Sum1 : Sum  SaturateOnIntegerOverflow=on
  y : Outport  InitialOutput=0
  wires:
  x/1 -> Sum/1
  Constant/1 -> Sum/2
  Sum/1 -> Product/1
  Constant1/1 -> Product/2
  Product/1 -> Gain/1
  Gain/1 -> Math Function/1
  Math Function/1 -> Sum1/1
  Constant2/1 -> Sum1/2
  Sum1/1 -> Math Function1/1
  Math Function1/1 -> y/1

== system neuronchainv5/Hebbconp/23/f(ui) ==
  x : Inport
  Constant : Constant  Value=offset
  Constant1 : Constant  Value=slope
  Constant2 : Constant
  Gain : Gain  Gain=-1  SaturateOnIntegerOverflow=on  OutDataTypeStr=Inherit: Same as input  ParamDataTypeStr=Inherit: Same as input
  Math Function : Math  SaturateOnIntegerOverflow=on
  Math Function1 : Math  Operator=reciprocal  SaturateOnIntegerOverflow=on
  Model Info : simulink/Model-Wide Utilities/Model Info  SystemSampleTime=-1  InitialBlockCM=None  BlockCM=None  Frame=on  DisplayStringWithTags=|  HorizontalTextAlignment=Center  LeftAlignmentValue=0.5  SourceBlockDiagram=neuronchainv5  TagMaxNumber=20
      | Model Info
      | %<Creator> Han, Cheol
  Product : Product  SaturateOnIntegerOverflow=on  OutDataTypeStr=Inherit: Same as first input
  Sum : Sum  Inputs=+-  SaturateOnIntegerOverflow=on
  Sum1 : Sum  SaturateOnIntegerOverflow=on
  y : Outport  InitialOutput=0
  wires:
  x/1 -> Sum/1
  Constant/1 -> Sum/2
  Sum/1 -> Product/1
  Constant1/1 -> Product/2
  Product/1 -> Gain/1
  Gain/1 -> Math Function/1
  Math Function/1 -> Sum1/1
  Constant2/1 -> Sum1/2
  Sum1/1 -> Math Function1/1
  Math Function1/1 -> y/1

== system neuronchainv5/Hebbconp/23/f(uj) ==
  x : Inport
  Constant : Constant  Value=offset
  Constant1 : Constant  Value=slope
  Constant2 : Constant
  Gain : Gain  Gain=-1  SaturateOnIntegerOverflow=on  OutDataTypeStr=Inherit: Same as input  ParamDataTypeStr=Inherit: Same as input
  Math Function : Math  SaturateOnIntegerOverflow=on
  Math Function1 : Math  Operator=reciprocal  SaturateOnIntegerOverflow=on
  Model Info : simulink/Model-Wide Utilities/Model Info  SystemSampleTime=-1  InitialBlockCM=None  BlockCM=None  Frame=on  DisplayStringWithTags=|  HorizontalTextAlignment=Center  LeftAlignmentValue=0.5  SourceBlockDiagram=neuronchainv5  TagMaxNumber=20
      | Model Info
      | %<Creator> Han, Cheol
  Product : Product  SaturateOnIntegerOverflow=on  OutDataTypeStr=Inherit: Same as first input
  Sum : Sum  Inputs=+-  SaturateOnIntegerOverflow=on
  Sum1 : Sum  SaturateOnIntegerOverflow=on
  y : Outport  InitialOutput=0
  wires:
  x/1 -> Sum/1
  Constant/1 -> Sum/2
  Sum/1 -> Product/1
  Constant1/1 -> Product/2
  Product/1 -> Gain/1
  Gain/1 -> Math Function/1
  Math Function/1 -> Sum1/1
  Constant2/1 -> Sum1/2
  Sum1/1 -> Math Function1/1
  Math Function1/1 -> y/1

== system neuronchainv5/Hebbconp/23/h(ui) ==
  x : Inport
  Constant : Constant  Value=offset
  Constant1 : Constant  Value=slope
  Constant2 : Constant
  Gain : Gain  Gain=-1  SaturateOnIntegerOverflow=on  OutDataTypeStr=Inherit: Same as input  ParamDataTypeStr=Inherit: Same as input
  Math Function : Math  SaturateOnIntegerOverflow=on
  Math Function1 : Math  Operator=reciprocal  SaturateOnIntegerOverflow=on
  Model Info : simulink/Model-Wide Utilities/Model Info  SystemSampleTime=-1  InitialBlockCM=None  BlockCM=None  Frame=on  DisplayStringWithTags=|  HorizontalTextAlignment=Center  LeftAlignmentValue=0.5  SourceBlockDiagram=neuronchainv5  TagMaxNumber=20
      | Model Info
      | %<Creator> Han, Cheol
  Product : Product  SaturateOnIntegerOverflow=on  OutDataTypeStr=Inherit: Same as first input
  Sum : Sum  Inputs=+-  SaturateOnIntegerOverflow=on
  Sum1 : Sum  SaturateOnIntegerOverflow=on
  y : Outport  InitialOutput=0
  wires:
  x/1 -> Sum/1
  Constant/1 -> Sum/2
  Sum/1 -> Product/1
  Constant1/1 -> Product/2
  Product/1 -> Gain/1
  Gain/1 -> Math Function/1
  Math Function/1 -> Sum1/1
  Constant2/1 -> Sum1/2
  Sum1/1 -> Math Function1/1
  Math Function1/1 -> y/1

== system neuronchainv5/Hebbconp/24/f(ui) ==
  x : Inport
  Constant : Constant  Value=offset
  Constant1 : Constant  Value=slope
  Constant2 : Constant
  Gain : Gain  Gain=-1  SaturateOnIntegerOverflow=on  OutDataTypeStr=Inherit: Same as input  ParamDataTypeStr=Inherit: Same as input
  Math Function : Math  SaturateOnIntegerOverflow=on
  Math Function1 : Math  Operator=reciprocal  SaturateOnIntegerOverflow=on
  Model Info : simulink/Model-Wide Utilities/Model Info  SystemSampleTime=-1  InitialBlockCM=None  BlockCM=None  Frame=on  DisplayStringWithTags=|  HorizontalTextAlignment=Center  LeftAlignmentValue=0.5  SourceBlockDiagram=neuronchainv5  TagMaxNumber=20
      | Model Info
      | %<Creator> Han, Cheol
  Product : Product  SaturateOnIntegerOverflow=on  OutDataTypeStr=Inherit: Same as first input
  Sum : Sum  Inputs=+-  SaturateOnIntegerOverflow=on
  Sum1 : Sum  SaturateOnIntegerOverflow=on
  y : Outport  InitialOutput=0
  wires:
  x/1 -> Sum/1
  Constant/1 -> Sum/2
  Sum/1 -> Product/1
  Constant1/1 -> Product/2
  Product/1 -> Gain/1
  Gain/1 -> Math Function/1
  Math Function/1 -> Sum1/1
  Constant2/1 -> Sum1/2
  Sum1/1 -> Math Function1/1
  Math Function1/1 -> y/1

== system neuronchainv5/Hebbconp/24/f(uj) ==
  x : Inport
  Constant : Constant  Value=offset
  Constant1 : Constant  Value=slope
  Constant2 : Constant
  Gain : Gain  Gain=-1  SaturateOnIntegerOverflow=on  OutDataTypeStr=Inherit: Same as input  ParamDataTypeStr=Inherit: Same as input
  Math Function : Math  SaturateOnIntegerOverflow=on
  Math Function1 : Math  Operator=reciprocal  SaturateOnIntegerOverflow=on
  Model Info : simulink/Model-Wide Utilities/Model Info  SystemSampleTime=-1  InitialBlockCM=None  BlockCM=None  Frame=on  DisplayStringWithTags=|  HorizontalTextAlignment=Center  LeftAlignmentValue=0.5  SourceBlockDiagram=neuronchainv5  TagMaxNumber=20
      | Model Info
      | %<Creator> Han, Cheol
  Product : Product  SaturateOnIntegerOverflow=on  OutDataTypeStr=Inherit: Same as first input
  Sum : Sum  Inputs=+-  SaturateOnIntegerOverflow=on
  Sum1 : Sum  SaturateOnIntegerOverflow=on
  y : Outport  InitialOutput=0
  wires:
  x/1 -> Sum/1
  Constant/1 -> Sum/2
  Sum/1 -> Product/1
  Constant1/1 -> Product/2
  Product/1 -> Gain/1
  Gain/1 -> Math Function/1
  Math Function/1 -> Sum1/1
  Constant2/1 -> Sum1/2
  Sum1/1 -> Math Function1/1
  Math Function1/1 -> y/1
